simulink model "task2_2"  (R2018a)
settings: Solver=ode4  StartTime=0.0  StopTime=simTime  FixedStep=sampleTime  RelTol=1e-3  EnableMultiTasking=on
InitFcn:
  | cd(fileparts(which(gcs)))
  | run ./initModel.m
StopFcn:
  | run ./postFcn.m;
values from neighbouring files (symbols this model uses):
  C = 1.5    [initModel.m]
  c0 = 21.3/2    (= 10.65)    [initModel.m]
  c1 = 1.11e-4    (= 0.000111)    [initModel.m]
  cLambda = 5.5e-1    (= 0.55)    [initModel.m]
  cPhi = 6e4    (= 60000)    [initModel.m]
  dwell = 0.5    [initModel.m]
  escK = 1875    [initModel.m]
  Fz0 = 4000    [initModel.m]
  g = 9.81    [initModel.m]
  h = 0.543    [initModel.m]
  h0 = h-(l1*h2+l2*h1)/L    (= 0.47616)    [initModel.m]
  h1 = 0.045    [initModel.m]
  h2 = 0.101    [initModel.m]
  Ixx = 1e3    (= 1000)    [initModel.m]
  Izz = 2617    [initModel.m]
  kLambda = 5.7e-1    (= 0.57)    [initModel.m]
  kPhi = 5e3    (= 5000)    [initModel.m]
  L = 2.675    [initModel.m]
  l1 = dist*L    (= 1.04325)    [initModel.m]
  l2 = L-l1    (= 1.63175)    [initModel.m]
  m = 1915    [initModel.m]
  ms = m-4e2    (= 1515)    [initModel.m]
  mu0 = 1    [initModel.m]
  mu1 = 6e-5    (= 6e-05)    [initModel.m]
  nst = 15.9    [initModel.m]
  rErrLim = 3e-1    (= 0.3)    [initModel.m]
  sampleTime = 0.01    [initModel.m]
  simTime = 100    [initModel.m]
  strAmpSS = 10    [initModel.m]
  strAmpSWD = 30    [initModel.m]
  strFreq = 0.7    [initModel.m]
  strMaxFreq = 20    [initModel.m]
  tStart = 1    [initModel.m]
  u0 = 100/3.6    (= 27.7777777778)    [initModel.m]
  uESCLim = 15/3.6    (= 4.16666666667)    [initModel.m]
  w = 1.6    [initModel.m]
libraries: simulink x1
settings Model: ExtModeAutoUpdateStatusClock=off  Creator=matthijs  LastModifiedBy=Abhishek B Bhat
settings DataIOCC: SaveFormat=Array  SignalLoggingSaveFormat=ModelDataLogs
settings OptimizationCC: ExpressionDepthLimit=2147483647  InitFltsAndDblsToZero=on  LifeSpan=inf
settings DebuggingCC: SaveWithParameterizedLinksMsg=none  UnderspecifiedInitializationDetection=Classic  MergeDetectMultiDrivingBlocksExec=none  SolverPrmCheckMsg=warning  MultiTaskCondExecSysMsg=none  FcnCallInpInsideContextMsg=warning  AllowSymbolicDim=off  StateNameClashWarn=warning  SFUnexpectedBacktrackingDiag=warning  SFNoUnconditionalDefaultTransitionDiag=warning  SFExecutionAtInitializationDiag=none
settings HardwareCC: ProdBitPerPointer=32  ProdBitPerSizeT=32  ProdBitPerPtrDiffT=32  ProdLargestAtomicFloat=None  ProdIntDivRoundTo=Undefined  ProdEndianess=Unspecified  ProdWordSize=32  ProdHWDeviceType=32-bit Generic
settings ModelReferenceCC: PropagateSignalLabelsOutOfModel=off
settings CodeAppCC: StateflowObjectComments=on
settings GRTTargetCC: TargetFcnLib=ansi_tfl_tmw.mat  TargetLangStandard=C89/C90 (ANSI)  GeneratePreprocessorConditionals=Disable all  CombineOutputUpdateFcns=off  GRTInterface=on
settings ConfigComp: CovMetricSettings=dw  CovHtmlReporting=on  CovSaveCumulativeToWorkspaceVar=on  CovSaveSingleToWorkspaceVar=on  CovExternalEMLEnable=off

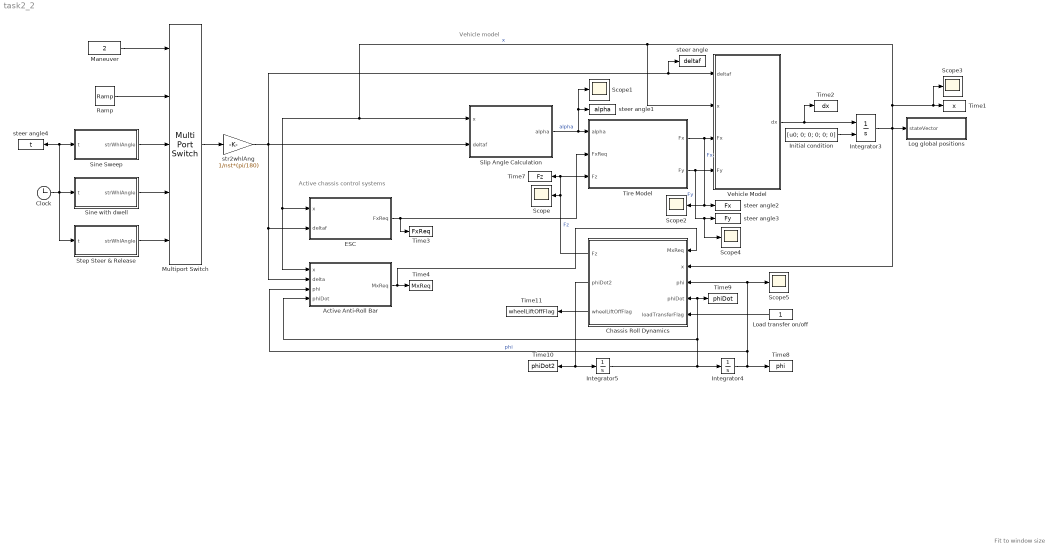
== system task2_2 ==
  note: Vehicle model
  note: Active chassis control systems
  note: Fit to window size
  Active Anti-Roll Bar : Subsystem
  Chassis Roll Dynamics : MATLAB Function  TreatAsAtomicUnit=on
  Clock : Clock
  ESC : Subsystem
  "Initial condition " : Constant  Value=[u0; 0; 0; 0; 0; 0]
  Integrator3 : Integrator  InitialConditionSource=external
  Integrator4 : Integrator
  Integrator5 : Integrator
  Load transfer on/off : Constant
  Log global positions : Subsystem
  Maneuver : Constant  Value=2
  Multiport Switch : MultiPortSwitch  Inputs=4
  Ramp : simulink/Sources/Ramp  slope=2e1  start=1  InitialOutput=0
  Scope{,1..5} (6 alike) : Scope
  Sine Sweep : Subsystem
  Sine with dwell : Subsystem
  Slip Angle Calculation : MATLAB Function  TreatAsAtomicUnit=on
  Step Steer & Release : Subsystem
  Time1 : ToWorkspace  VariableName=x  SampleTime=sampleTime
  Time10 : ToWorkspace  VariableName=phiDot2  SampleTime=sampleTime
  Time11 : ToWorkspace  VariableName=wheelLiftOffFlag  SampleTime=sampleTime
  Time2 : ToWorkspace  VariableName=dx  SampleTime=sampleTime
  Time3 : ToWorkspace  VariableName=FxReq  SampleTime=sampleTime
  Time4 : ToWorkspace  VariableName=MxReq  SampleTime=sampleTime
  Time7 : ToWorkspace  VariableName=Fz  SampleTime=sampleTime
  Time8 : ToWorkspace  VariableName=phi  SampleTime=sampleTime
  Time9 : ToWorkspace  VariableName=phiDot  SampleTime=sampleTime
  Tire Model : MATLAB Function  TreatAsAtomicUnit=on
  Vehicle Model : MATLAB Function  TreatAsAtomicUnit=on
  steer angle : ToWorkspace  VariableName=deltaf  SampleTime=sampleTime
  steer angle1 : ToWorkspace  VariableName=alpha  SampleTime=sampleTime
  steer angle2 : ToWorkspace  VariableName=Fx  SampleTime=sampleTime
  steer angle3 : ToWorkspace  VariableName=Fy  SampleTime=sampleTime
  steer angle4 : ToWorkspace  VariableName=t  SampleTime=sampleTime
  str2whlAng : Gain  Gain=1/nst*(pi/180)
  wires:
  Slip Angle Calculation/1(alpha) -> Scope1/1, steer angle1/1, Tire Model/1(alpha)  "alpha"
  Integrator3/1 -> Slip Angle Calculation/1(x), Active Anti-Roll Bar/1(x), ESC/1(x), Vehicle Model/2(x), Scope3/1, Time1/1, Log global positions/1(stateVector), Chassis Roll Dynamics/2(x)  "x"
  Vehicle Model/1(dx) -> Time2/1, Integrator3/1
  Tire Model/2(Fy) -> Vehicle Model/4(Fy), Scope4/1, steer angle3/1  "Fy"
  Tire Model/1(Fx) -> Scope2/1, steer angle2/1, Vehicle Model/3(Fx)  "Fx"
  Chassis Roll Dynamics/2(phiDot2) -> Integrator5/1, Time10/1
  Integrator5/1 -> Integrator4/1, Active Anti-Roll Bar/4(phiDot), Time9/1, Chassis Roll Dynamics/4(phiDot)
  Integrator4/1 -> Chassis Roll Dynamics/3(phi), Scope5/1, Active Anti-Roll Bar/3(phi), Time8/1  "phi"
  ESC/1(FxReq) -> Tire Model/2(FxReq), Time3/1
  Chassis Roll Dynamics/3(wheelLiftOffFlag) -> Time11/1
  Clock/1 -> Sine Sweep/1(t), steer angle4/1, Step Steer & Release/1(t), Sine with dwell/1(t)
  Load transfer on/off/1 -> Chassis Roll Dynamics/5(loadTransferFlag)
  Active Anti-Roll Bar/1(MxReq) -> Chassis Roll Dynamics/1(MxReq), Time4/1
  "Initial condition "/1 -> Integrator3/2
  str2whlAng/1 -> Active Anti-Roll Bar/2(delta), ESC/2(deltaf), steer angle/1, Vehicle Model/1(deltaf), Slip Angle Calculation/2(deltaf)
  Multiport Switch/1 -> str2whlAng/1
  Chassis Roll Dynamics/1(Fz) -> Time7/1, Tire Model/3(Fz), Scope/1  "Fz"
  Step Steer & Release/1(strWhlAngle) -> Multiport Switch/5
  Sine with dwell/1(strWhlAngle) -> Multiport Switch/4
  Sine Sweep/1(strWhlAngle) -> Multiport Switch/3
  Maneuver/1 -> Multiport Switch/1
  Ramp/1 -> Multiport Switch/2

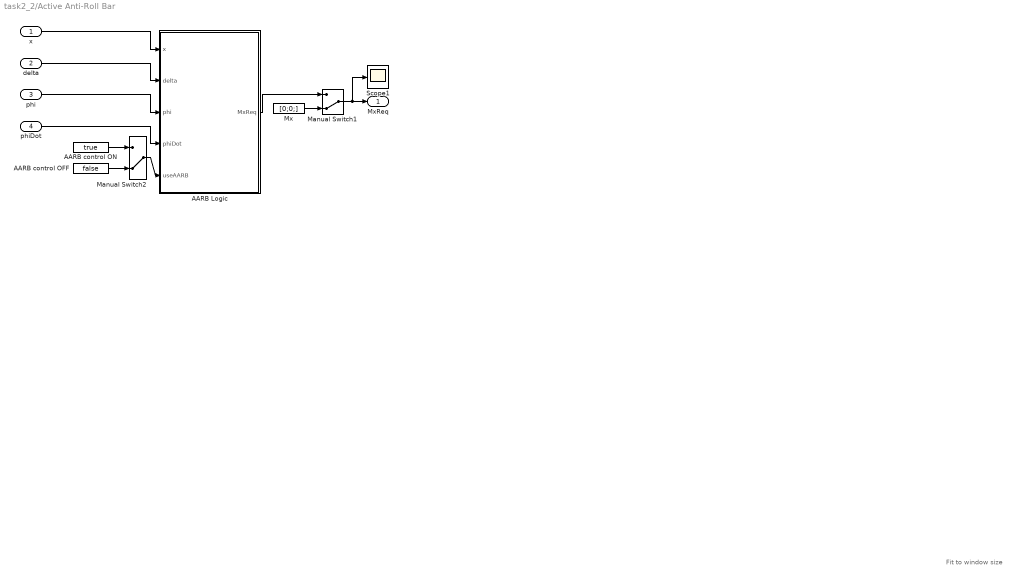
== system task2_2/Active Anti-Roll Bar ==
  note: Fit to window size
  x : Inport
  delta : Inport  Port=2
  phi : Inport  Port=3
  phiDot : Inport  Port=4
  AARB Logic : MATLAB Function  TreatAsAtomicUnit=on
  AARB control OFF : Constant  Value=false
  AARB control ON : Constant  Value=true
  Manual Switch1 : ManualSwitch  CurrentSetting=0
  Manual Switch2 : ManualSwitch  CurrentSetting=0
  Mx : Constant  Value=[0;0;]
  Scope1 : Scope
  MxReq : Outport
  wires:
  Mx/1 -> Manual Switch1/2
  Manual Switch1/1 -> MxReq/1, Scope1/1
  AARB control ON/1 -> Manual Switch2/1
  AARB control OFF/1 -> Manual Switch2/2
  Manual Switch2/1 -> AARB Logic/5(useAARB)
  AARB Logic/1(MxReq) -> Manual Switch1/1
  phi/1 -> AARB Logic/3(phi)
  phiDot/1 -> AARB Logic/4(phiDot)
  x/1 -> AARB Logic/1(x)
  delta/1 -> AARB Logic/2(delta)

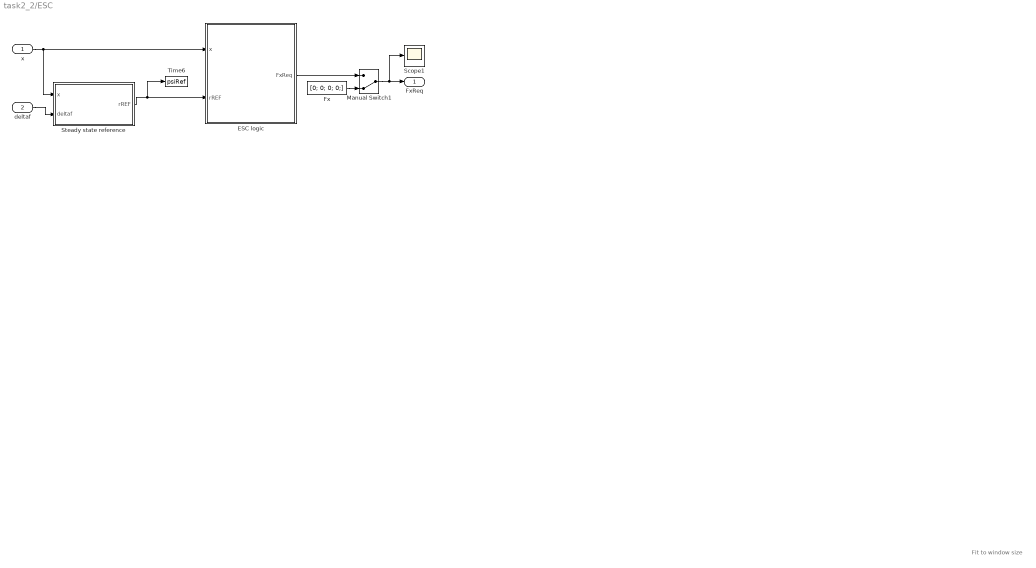
== system task2_2/ESC ==
  note: Fit to window size
  x : Inport
  deltaf : Inport  Port=2
  ESC logic : MATLAB Function  TreatAsAtomicUnit=on
  Fx : Constant  Value=[0; 0; 0; 0;]
  Manual Switch1 : ManualSwitch  CurrentSetting=0
  Scope1 : Scope
  Steady state reference : MATLAB Function  TreatAsAtomicUnit=on
  Time6 : ToWorkspace  VariableName=psiRef  SampleTime=sampleTime
  FxReq : Outport
  wires:
  deltaf/1 -> Steady state reference/2(deltaf)
  Manual Switch1/1 -> FxReq/1, Scope1/1
  Fx/1 -> Manual Switch1/2
  ESC logic/1(FxReq) -> Manual Switch1/1
  x/1 -> Steady state reference/1(x), ESC logic/1(x)
  Steady state reference/1(rREF) -> Time6/1, ESC logic/2(rREF)

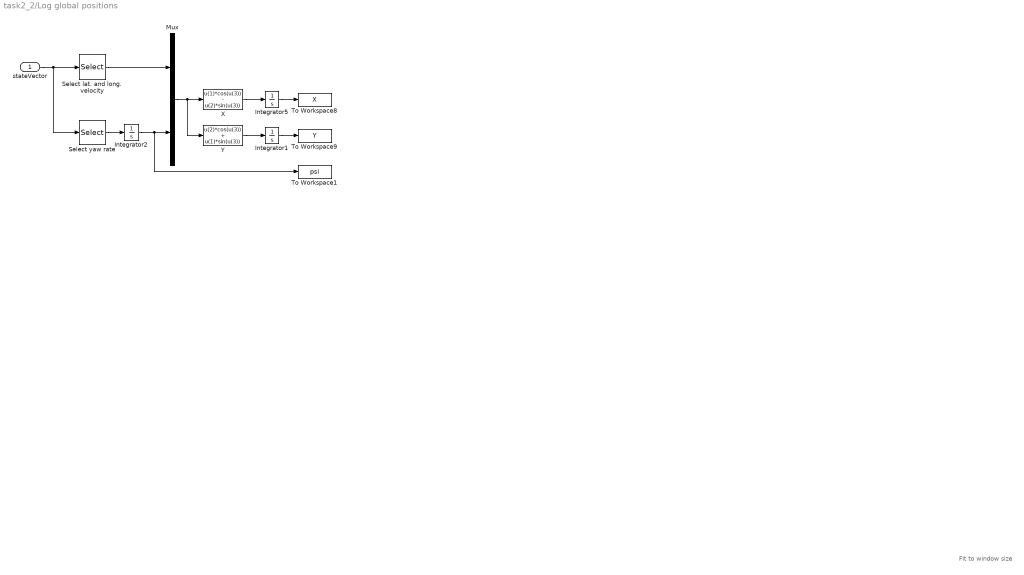
== system task2_2/Log global positions ==
  note: Fit to window size
  stateVector : Inport
  Integrator1 : Integrator
  Integrator2 : Integrator
  Integrator5 : Integrator
  Mux : Mux  Inputs=2
  Select yaw rate : Selector  InputPortWidth=6  IndexOptions=Index vector (dialog)  Indices=3  OutputSizes=1
  Select lat. and long. velocity : Selector  InputPortWidth=6  IndexOptions=Index vector (dialog)  Indices=[1 2]  OutputSizes=1
  To Workspace1 : ToWorkspace  VariableName=psi  SampleTime=sampleTime
  To Workspace8 : ToWorkspace  VariableName=X  SampleTime=sampleTime
  To Workspace9 : ToWorkspace  VariableName=Y  SampleTime=sampleTime
  X : Fcn  Expr=u(1)*cos(u(3)) - u(2)*sin(u(3))
  Y : Fcn  Expr=u(2)*cos(u(3)) + u(1)*sin(u(3))
  wires:
  Select yaw rate/1 -> Integrator2/1
  Select lat. and long. velocity/1 -> Mux/1
  Integrator2/1 -> To Workspace1/1, Mux/2
  Mux/1 -> X/1, Y/1
  X/1 -> Integrator5/1
  Y/1 -> Integrator1/1
  stateVector/1 -> Select yaw rate/1, Select lat. and long. velocity/1
  Integrator5/1 -> To Workspace8/1
  Integrator1/1 -> To Workspace9/1

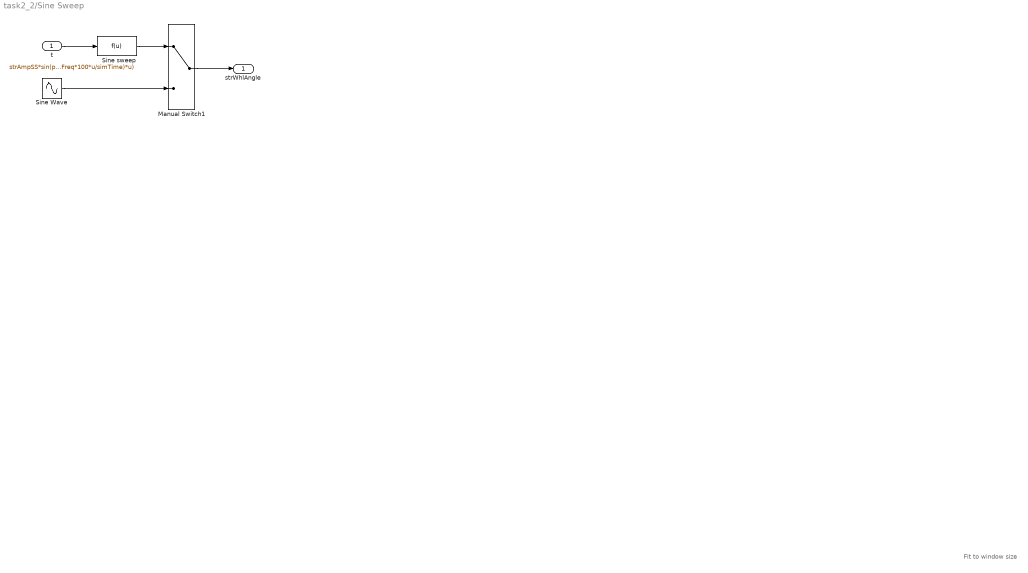
== system task2_2/Sine Sweep ==
  note: Fit to window size
  t : Inport
  Manual Switch1 : ManualSwitch
  Sine Wave : Sin  Amplitude=strAmpSS  Frequency=strMaxFreq*2*pi  SampleTime=0
  Sine sweep : Fcn  Expr=strAmpSS*sin(pi*(strMaxFreq*100*u/simTime)*u)
  strWhlAngle : Outport
  wires:
  t/1 -> Sine sweep/1
  Sine Wave/1 -> Manual Switch1/2
  Manual Switch1/1 -> strWhlAngle/1
  Sine sweep/1 -> Manual Switch1/1

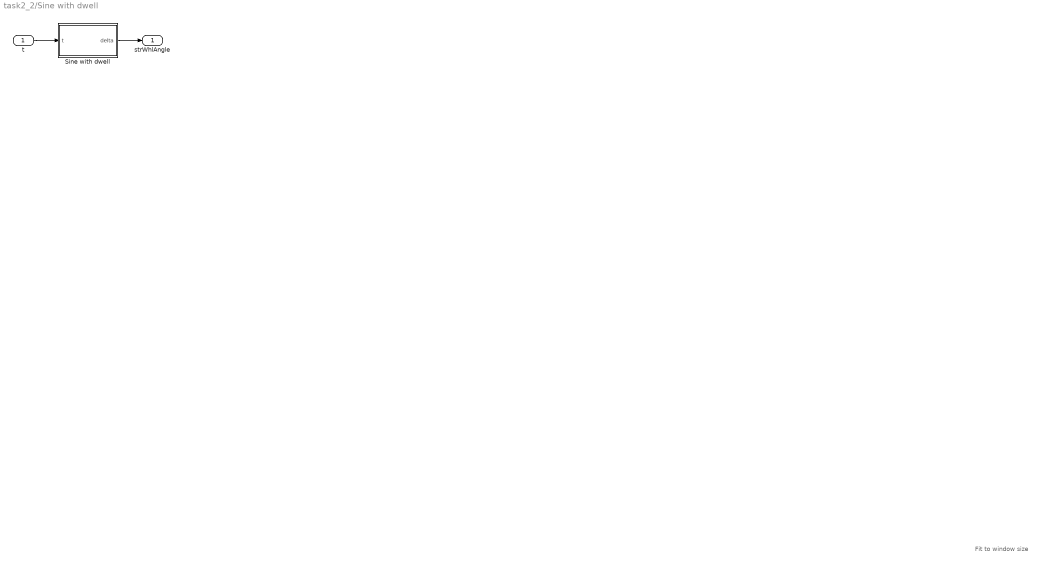
== system task2_2/Sine with dwell ==
  note: Fit to window size
  t : Inport
  Sine with dwell : MATLAB Function  TreatAsAtomicUnit=on
  strWhlAngle : Outport
  wires:
  t/1 -> Sine with dwell/1(t)
  Sine with dwell/1(delta) -> strWhlAngle/1

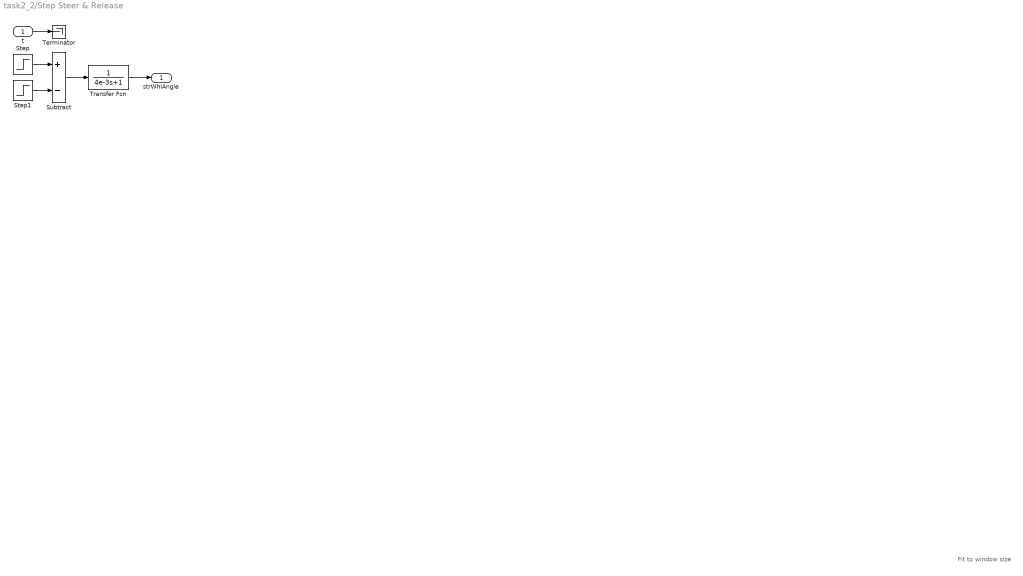
== system task2_2/Step Steer & Release ==
  note: Fit to window size
  t : Inport
  Step : Step  After=strAmpSS  SampleTime=0
  Step1 : Step  Time=6  After=strAmpSS  SampleTime=0
  Subtract : Sum  Inputs=+-
  Terminator : Terminator
  Transfer Fcn : TransferFcn  Denominator=[4e-3 1]
  strWhlAngle : Outport
  wires:
  Transfer Fcn/1 -> strWhlAngle/1
  t/1 -> Terminator/1
  Step/1 -> Subtract/1
  Subtract/1 -> Transfer Fcn/1
  Step1/1 -> Subtract/2

== matlab function task2_2/Vehicle Model ==
  settings: fimath=|
      | fimath(...
      | 'RoundMode', 'floor',...
      | 'OverflowMode', 'wrap',...
      | 'ProductMode', 'KeepLSB', 'ProductWordLength', 32,...
      | 'SumMode', 'KeepLSB', 'SumWordLength', 32,...
      | 'CastBeforeSum', false)
  data: dx output; deltaf input; x input; Fx input; Fy input; m parameter; Izz parameter; l1 parameter; l2 parameter; w parameter; sampleTime parameter
%% --------------------------------------------------------------------- %%
function dx = EqnsOfMotion(deltaf,x,Fx,Fy,m,Izz,l1,l2,w,sampleTime)
    % Input: Vector of vehicle states (x), road wheel angle (deltaf),
    % vector of lateral and longitudinal wheel forces (Fy and Fx), vehicle
    % parameters
    % Output: Derivative of vector of vehicle states (dx)
    %%===================================================================%%
    % x = [Long. vel; Lat vel; Yaw rate; Long acc; Lat acc; Yaw acc]
    vx  = x(1);
    vy  = x(2);
    r   = x(3);
    dx  = zeros(6,1);
    %%===================================================================%%
    % Equations of motion
    dvx = (((Fx(1)+Fx(2))*cos(deltaf)-(Fy(1)+Fy(2))*sin(deltaf)+Fx(3)+Fx(4))/m)+(r*vy);;
    dvy = (((Fx(1)+Fx(2))*sin(deltaf)+(Fy(1)+Fy(2))*cos(deltaf)+Fy(3)+Fy(4))/m)-(r*vx);
    dr  = (((Fx(1)+Fx(2))*sin(deltaf)+(Fy(1)+Fy(2))*cos(deltaf))*l1-(Fy(3)+Fy(4))*l2-....
                    (Fx(1)*cos(deltaf)-Fx(2)*cos(deltaf)-Fy(1)*sin(deltaf)+Fy(2)*sin(deltaf)+Fx(3)-Fx(4))*(w/2))/Izz;
    %%===================================================================%%
    % State derivatives
    dx(1:3) = [dvx; dvy; dr;];
    % Creating extra state derivates
    dx(4)   = (dvx-r*vy - x(4))/sampleTime;
    dx(5)   = (dvy+r*vx - x(5))/sampleTime;
    dx(6)   = (dr - x(6))/sampleTime;
    % These extra state derivates, when integrated give ax, ay and r_dot.
    % This is done in order to overcome an algebraic loop problem (i.e,
    % load transfer depends on accelerations which depend on tyre forces
    % which depend on load transfer again -> a chicken and an egg problem).
end
% end of file

== matlab function task2_2/Chassis Roll Dynamics ==
  data: MxReq input; x input; phi input; phiDot input; Fz output; m parameter; phiDot2 output; wheelLiftOffFlag output; ms parameter; Ixx parameter; l1 parameter; l2 parameter; L parameter; w parameter; h parameter; h0 parameter; h1 parameter; h2 parameter; g parameter; cPhi parameter; cLambda parameter; kPhi parameter; kLambda parameter; loadTransferFlag input
%% --------------------------------------------------------------------- %%
function [Fz,phiDot2,wheelLiftOffFlag] = LoadTransfer(MxReq,x,phi,...
    phiDot,m,ms,Ixx,l1,l2,L,w,h,h0,h1,h2,g,cPhi,cLambda,kPhi,kLambda,...
    loadTransferFlag)
    % Inputs: Vehicle states (x), roll angle and roll rate (phi, phiDot),
    % vehicle parameters
    % Outputs: Wheel normal loads (Fz), roll acceleration (phiDDot), flag
    % indicating wheel lift-off (wheelLiftOffFlag)
    %%===================================================================%%
    ax       = x(4);
    ay       = x(5);
    MxExtFr  = MxReq(1);
    MxExtRe  = MxReq(2);
    %
    % Dummy Fz values -> Change them accordingly
FzStatic = ((m*g)/(L*2))*[l2;l2;l1;l1];

    %%===================================================================%%
    % Dynamic load transfer for roll and steady state load transfer for 
    % pitch motion

cPhi1   = cPhi*cLambda;
cPhi2   = cPhi - cPhi1;
kPhi1   = kPhi*kLambda;
kPhi2   = kPhi - kPhi1;
    

dFzy = [+((m*(l2)*ay*h1)/L + cPhi1*phi + kPhi1*phiDot +MxExtFr/2)/w;
        -((m*(l2)*ay*h1)/L + cPhi1*phi + kPhi1*phiDot +MxExtFr/2)/w;
        +((m*(l1)*ay*h2)/L + cPhi2*phi + kPhi2*phiDot +MxExtRe/2)/w;  
        -((m*(l1)*ay*h2)/L + cPhi2*phi + kPhi2*phiDot +MxExtRe/2)/w];

dFzx = [-m*ax*h/(2*L);
        -m*ax*h/(2*L);
        +m*ax*h/(2*L);
        +m*ax*h/(2*L)];
    Fz      = FzStatic + dFzx*loadTransferFlag + dFzy*loadTransferFlag;
    
phiDot2 = (ms*ay*h0 - kPhi*phiDot - (cPhi - ms*g*h0)*phi - MxExtFr -MxExtRe)/(Ixx + ms*h0^2);

    %%===================================================================%%
    % % Wheel lift-off scenario. This is not really *handling* wheel lift-,
    % off but rather making sure the simulation does not crash in the event
    % of wheel lift-off. Solution may still be incorrect. Handling wheel
    % lift-off is not straight forward. So this simulation model is not
    % good for cases with excessive or frequent wheel lift-off.
    eps              = 1e-2;
    wheelLiftOffFlag = 0;
    if any(Fz < 0) 
        wheelLiftOffFlag = 1;
    else
            wheelLiftOffFlag = 0;
    end
    Fz(Fz < eps) = eps;
end
% end of file

== matlab function task2_2/Slip Angle Calculation ==
  settings: fimath=|
      | fimath(...
      | 'RoundMode', 'floor',...
      | 'OverflowMode', 'wrap',...
      | 'ProductMode', 'KeepLSB', 'ProductWordLength', 32,...
      | 'SumMode', 'KeepLSB', 'SumWordLength', 32,...
      | 'CastBeforeSum', false)
  data: alpha output; x input; deltaf input; l1 parameter; l2 parameter; w parameter
%% --------------------------------------------------------------------- %%
function alpha = SlipAngles(x,deltaf,l1,l2,w) 
    % Inputs: Vector of vehicle states (x), road wheel angle (deltaf) and
    % vehicle parameters
    % Output: alpha is the vector of slip angles of the 4 tyres
    %%===================================================================%%
    vx    = x(1);
    vy    = x(2);
    r     = x(3);
    %%===================================================================%%
    alpha_1 = -atan((vy+l1*r)/(vx - (w*r/2))) + deltaf;
    alpha_2 = -atan((vy+l1*r)/(vx + (w*r/2))) + deltaf;
    alpha_3 = -atan((vy-l2*r)/(vx - (w*r/2)));
    alpha_4 = -atan((vy-l2*r)/(vx + (w*r/2)));
    alpha = [alpha_1, alpha_2, alpha_3, alpha_4;]';
end
% end of file

== matlab function task2_2/Active Anti-Roll Bar/AARB Logic ==
  data: x input; delta input; MxReq output; phi input; phiDot input; useAARB input; cPhi parameter; kPhi parameter; cLambda parameter; kLambda parameter; h parameter; h1 parameter; h2 parameter; l1 parameter; l2 parameter; L parameter; m parameter
%% --------------------------------------------------------------------- %%
function MxReq = AARB_Control(x,delta,phi,phiDot,useAARB,cPhi,kPhi,...
    cLambda,kLambda,h, h1, h2, l1, l2, L,m)
% Active anti roll bar torque request
MxReq = [0; 0];

%reference roll angle 
deltaH = h-((l2*h1+l1*h2)/L);
target_roll= (m*x(5)*deltaH)/cPhi ;

K_gain = 12;
if phi>0
            ref_err = target_roll - phi;
            roll_err_abs= 100*abs(ref_err/target_roll);
            Mxf = K_gain*roll_err_abs;
            Mxr = K_gain*roll_err_abs;
            
            MxReq = [Mxf; Mxr];
elseif phi<0
            ref_err = target_roll - phi;
            roll_err_abs= 100*abs(ref_err/target_roll);
            Mxf = -K_gain*roll_err_abs;
            Mxr = -K_gain*roll_err_abs;
            MxReq = [Mxf; Mxr];
end
% end of file

== matlab function task2_2/Sine with dwell/Sine with dwell ==
  data: delta output; t input; tStart parameter; strAmpSWD parameter; dwell parameter; strFreq parameter
function delta = SWD(t,tStart,strAmpSWD,dwell,strFreq)

t0  = tStart;
A   = strAmpSWD;
f   = strFreq;

T=1/f;

if t > t0 && t <= t0 + 3*T/4
    delta = A*sin(2*pi*f*(t - t0));
elseif t > t0 + 3*T/4 && t <= t0 + 3*T/4 + dwell
    delta = A*sin(2*pi*f*(3*T/4));
elseif t > t0 + 3*T/4 + dwell && t <= t0 + T + dwell 
    delta = A*sin(2*pi*f*(t - (t0 + dwell)));
else
    delta = 0;    
end

== matlab function task2_2/ESC/ESC logic ==
  data: x input; rREF input; FxReq output; escK parameter; rErrLim parameter; uESCLim parameter
%% --------------------------------------------------------------------- %%
function FxReq = StabilityControl(x,rREF,escK,rErrLim,uESCLim)
vx = x(1);
r  = x(3);
%-------------------------------- ESC --------------------------------%
% Longitudinal force request
FxReq = [0; 0; 0; 0;];
min_r = 0.01;

if (vx>uESCLim)
    if rREF > 0
        if r < 0
            r_err = rREF - r;
            r_err_perc = 100*abs(r_err/rREF);
            
            Fx1 = escK*r_err_perc;
            FxReq = [-Fx1;0;0;0];
            
        elseif r > 0
            if abs(rREF) >= min_r
                
                r_err = r - rREF;
                r_err_perc = 100*abs(r_err/rREF);
                
                if r_err < 0 && r_err_perc >= rErrLim
                    Fx3 = escK*r_err_perc;
                    FxReq = [0;0;-Fx3;0];
                    
                elseif r_err > 0 && r_err_perc >= rErrLim
                    Fx2 = escK*r_err_perc;
                    FxReq = [0;-Fx2;0;0];
                end
            end
        end
        
        
    elseif rREF < 0
        if r > 0
            r_err = rREF - r;
            r_err_perc = 100*abs(r_err/rREF);
            
            Fx2 = escK*r_err_perc;
            FxReq = [0;-Fx2;0;0];
            
            
        elseif r < 0
            if abs(rREF) >= min_r
                
                r_err = r - rREF;
                r_err_perc = 100*abs(r_err/rREF);
                
                if r_err > 0 && r_err_perc >= rErrLim
                    Fx4 = escK*r_err_perc;
                    FxReq = [0;0;0;-Fx4];
                    
                elseif r_err < 0 && r_err_perc >= rErrLim
                    Fx1 = escK*r_err_perc;
                    FxReq = [-Fx1;0;0;0];
                end
            end
        end
    elseif r == 0 && rREF ~= 0
        r_err = r;
        r_err_perc = 100*abs(r_err);
        
        if r_err <= 0 && r_err_perc >= rErrLim
            Fx1 = escK*r_err_perc;
            FxReq = [-Fx1;0;0;0];
            
        elseif r_err > 0 && r_err_perc >= rErrLim
            Fx2 = escK*r_err_perc;
            FxReq = [0;-Fx2;0;0];
        end
    end
end
end

== matlab function task2_2/Tire Model ==
  settings: fimath=|
      | fimath(...
      | 'RoundMode', 'floor',...
      | 'OverflowMode', 'wrap',...
      | 'ProductMode', 'KeepLSB', 'ProductWordLength', 32,...
      | 'SumMode', 'KeepLSB', 'SumWordLength', 32,...
      | 'CastBeforeSum', false)
  data: Fx output; alpha input; FxReq input; Fz input; Fy output; C parameter; E parameter; mu0 parameter; mu1 parameter; c0 parameter; c1 parameter; Fz0 parameter
%% --------------------------------------------------------------------- %%
function [Fx,Fy]= MagicTireEq(alpha,FxReq,Fz,C,E,mu0,mu1,c0,c1,Fz0)
    % Input: Vector of slip angles (alpha), Fx request from the ESC
    % controller (FxReq), normal load on the tyres (Fz)
    % Output: Vector of lateral forces of the 4 tyres (Fy) and vector or
    % longitudinal forces of the 4 tyres (Fx)
    %%===================================================================%%
    mu = mu0*(1-mu1*(Fz-Fz0));
    c  = c0*(1-c1*(Fz-Fz0));
    B  = c./(mu*C);
    %%===================================================================%%
    % Force limitation and combined slip
    Fx_t = [0 0 0 0];
    
for i = 1:4
    if mu(i)*Fz(i) < FxReq(i)
        Fx_t(i) = mu(i).*Fz(i);
    elseif FxReq(i) < -mu(i)*Fz(i)*cos(alpha(i))
        Fx_t(i) = -mu(i)*Fz(i)*cos(alpha(i));
    end
end
    Fx    = [Fx_t(1), Fx_t(2), Fx_t(3), Fx_t(4);]';
    
    Fymax_t = [0 0 0 0];
    
    for i=1:4
    Fymax_t(i) = sqrt(((mu(i)*Fz(i))^2)-Fx(i)^2);
    end
    FyMax = [Fymax_t(1), Fymax_t(2), Fymax_t(3), Fymax_t(4);]';
    %%===================================================================%%
    Fy    = FyMax.*sin(C*atan(B.*alpha-E*(B.*alpha-atan(B.*alpha))));
end
% end of file

== matlab function task2_2/ESC/Steady state reference ==
  data: x input; deltaf input; rREF output; c0 parameter; c1 parameter; Fz0 parameter; m parameter; l1 parameter; l2 parameter; L parameter; g parameter; mu0 parameter; mu1 parameter; C parameter; E parameter
%% --------------------------------------------------------------------- %%
function rREF = RefGen(x,deltaf,c0,c1,Fz0,m,l1,l2,L,g,mu0,mu1, C, E)
%% cornering stiffness
   g = 9.81;
Fz0_init = (m*g/(2*L))  *[l2; l2; l1; l1];
mu_init      = mu0*(1-mu1*(Fz0_init-Fz0));
c_init       = c0*(1-c1*(Fz0_init-Fz0));
B_init       = c_init./(mu_init*C);

FyMax_init  = mu_init.*Fz0_init;

alpha0 = 0.001;
Fy1_init = FyMax_init.*sin(C*atan(B_init.*alpha0-E*(B_init.*alpha0-atan(B_init.*alpha0))));
Ci_init = Fy1_init/alpha0;

Cf_nl = Ci_init(1) + Ci_init(2);
Cr_nl = Ci_init(3) + Ci_init(4);
C_nl = [Cf_nl; Cr_nl];

    % Parameters
vx = x(1);

   % Reference yaw rate
   
rDES = (C_nl(1)*C_nl(2)*L*vx*deltaf)/(C_nl(1)*C_nl(2)*L^2-m*(vx^2)*(C_nl(1)*l1-C_nl(2)*l2));
mu = 0.9 % 0.9 limit
r_max = abs(mu*g/vx);

if rDES > r_max
    rREF = r_max;
elseif rDES < -r_max
    rREF = -r_max;
else
    rREF = rDES;
end
   

end
%end of file
